simulink model "bijiao"  (R2022b)
settings: Solver=VariableStepAuto  StartTime=0.0  StopTime=50  RelTol=1e-3
settings Model: Creator=HONOR  LastModifiedBy=acer
settings DebuggingCC: UnconnectedInputMsg=warning  UnconnectedOutputMsg=warning  UnconnectedLineMsg=warning
settings ModelReferenceCC: EnableRefExpFcnMdlSchedulingChecks=on
settings RTWCC: DLArmComputeVersion=19.05

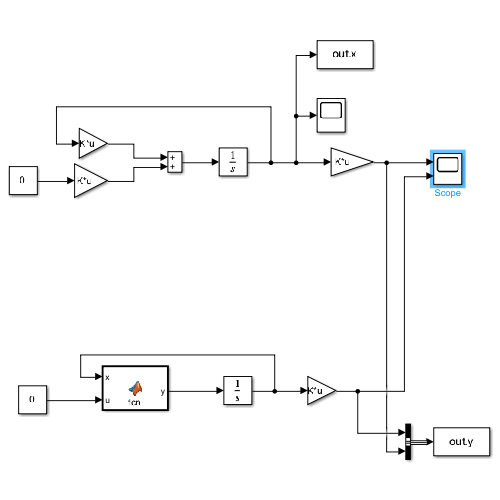
[thumbnail: Simulink's stored preview of the top-level diagram]
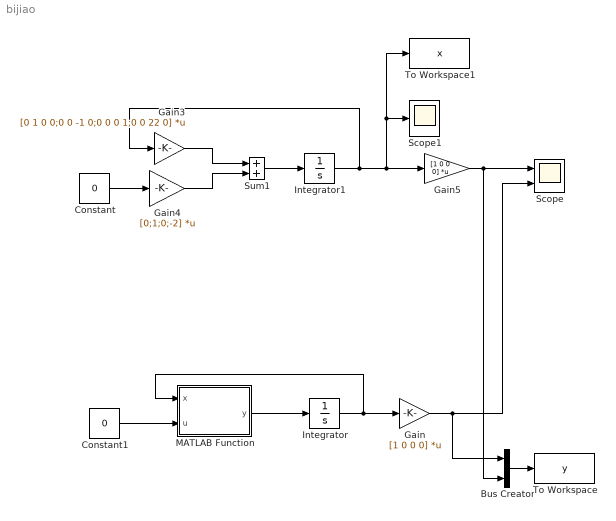
== system bijiao ==
  Bus Creator : BusCreator  Inputs=2
  Constant : Constant  Value=0
  Constant1 : Constant  Value=0
  Gain : Gain  Gain=[1 0 0 0]  Multiplication=Matrix(K*u)
  Gain3 : Gain  Gain=[0 1 0 0;0 0 -1 0;0 0 0 1;0 0 22 0]  Multiplication=Matrix(K*u)
  Gain4 : Gain  Gain=[0;1;0;-2]  Multiplication=Matrix(K*u)
  Gain5 : Gain  Gain=[1 0 0 0]  Multiplication=Matrix(K*u)
  Integrator : Integrator  InitialCondition=[0,0,0.1,0]
  Integrator1 : Integrator  InitialCondition=[0,0,0.1,0]
  MATLAB Function : MATLAB Function  TreatAsAtomicUnit=on
  Scope : Scope  NumInputPorts=2
  Scope1 : Scope
  Sum1 : Sum
  To Workspace : ToWorkspace  VariableName=y  SaveFormat=Structure With Time  SampleTime=-1
  To Workspace1 : ToWorkspace  VariableName=x  SaveFormat=Structure With Time  SampleTime=-1
  wires:
  Constant/1 -> Gain4/1
  Gain5/1 -> Bus Creator/2, Scope/1
  Gain3/1 -> Sum1/1
  Gain4/1 -> Sum1/2
  Sum1/1 -> Integrator1/1
  Integrator1/1 -> Gain5/1, To Workspace1/1, Scope1/1, Gain3/1
  Constant1/1 -> MATLAB Function/2(u)
  MATLAB Function/1(y) -> Integrator/1
  Integrator/1 -> MATLAB Function/1(x), Gain/1
  Gain/1 -> Bus Creator/1, Scope/2
  Bus Creator/1 -> To Workspace/1

== matlab function bijiao/MATLAB Function ==
  data: x input; u input; y output
function y = fcn(x, u)
M=1;
m=0.1;
l=0.5;
g=10;
Dx3=x(4);
Dx4=(u*cos(x(3))-(M+m)*g*sin(x(3))+m*l*sin(x(3))*cos(x(3)*x(4)))/(m*l*cos(x(3))*cos(x(3))-(M+m)*l);
Dx1=x(2);
Dx2=((u+m*l*sin(x(3)*x(4)*x(4))-m*g*cos(x(3))*sin(x(3)))/(M+m-m*cos(x(3))*cos(x(3))));
y=[Dx1;Dx2;Dx3;Dx4];
